simulink model "ControlSystems19"  (R2020b)
settings: Solver=VariableStepAuto  StartTime=0.0  StopTime=100  FixedStep=0.001  MinStep=1e-5
undefined symbols (not defined in the file): DiscIntNeverNeededParam, magnitude
libraries: fl_lib x8, ee_lib x6, nesl_utility x6, pid_lib x5, simulink x3, powerlib x1
(part 1 of 2)
settings Model: Creator=markb  LastModifiedBy=orangejuzi
settings SolverCC: ShapePreserveControl=EnableAll  AlgebraicLoopSolver=LineSearch  MinimalZcImpactIntegration=on
settings DebuggingCC: ReadBeforeWriteMsg=DisableAll  WriteAfterWriteMsg=DisableAll  WriteAfterReadMsg=DisableAll  MaxConsecutiveZCsMsg=warning  MultiTaskDSMMsg=none  ModelReferenceExtraNoncontSigs=warning
settings ModelReferenceCC: UpdateModelReferenceTargets=IfOutOfDate
settings SFSimCC: SFSimEcho=off

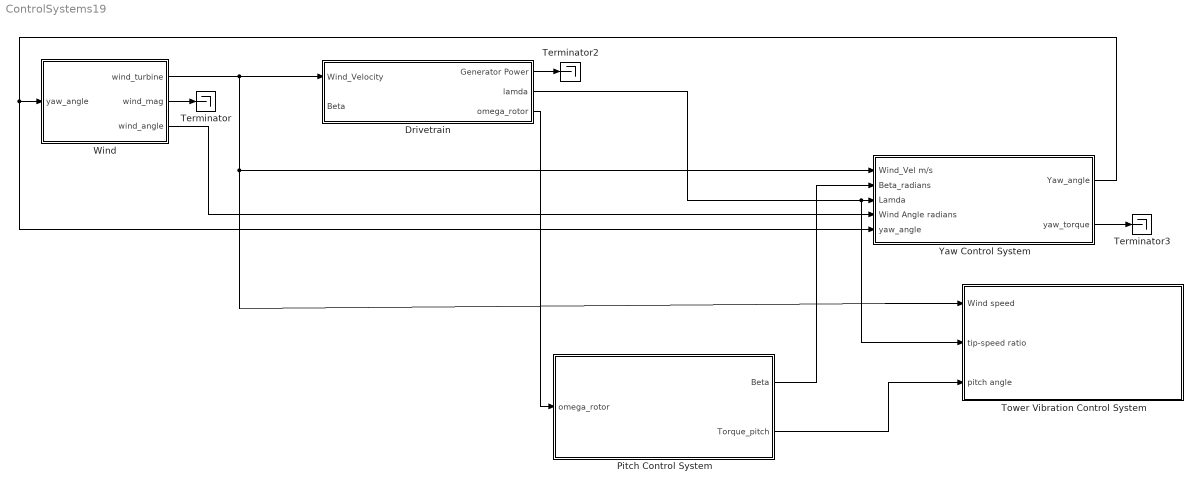
== system ControlSystems19 ==
  Drivetrain : Subsystem
  Pitch Control System : Subsystem
  Terminator : Terminator
  Terminator2 : Terminator
  Terminator3 : Terminator
  Tower Vibration Control System : Subsystem
  Wind : Subsystem
  Yaw Control System : Subsystem
  wires:
  Yaw Control System/1(Yaw_angle) -> Yaw Control System/5(yaw_angle), Wind/1(yaw_angle)
  Wind/2(wind_mag) -> Terminator/1
  Drivetrain/1(Generator Power) -> Terminator2/1
  Wind/3(wind_angle) -> Yaw Control System/4(Wind Angle radians)
  Wind/1(wind_turbine) -> Drivetrain/1(Wind_Velocity), Tower Vibration Control System/1(Wind speed), Yaw Control System/1(Wind_Vel m/s)
  Yaw Control System/2(yaw_torque) -> Terminator3/1
  Drivetrain/2(lamda) -> Tower Vibration Control System/2(tip-speed ratio), Yaw Control System/3(Lamda)
  Drivetrain/3(omega_rotor) -> Pitch Control System/1(omega_rotor)
  Pitch Control System/1(Beta) -> Yaw Control System/2(Beta_radians)
  Pitch Control System/2(Torque_pitch) -> Tower Vibration Control System/3("pitch angle ")

== system ControlSystems19/Drivetrain ==
  Wind_Velocity : Inport
  Beta : Inport  Port=2
  Aerodynamic Block : Subsystem
  Electricl Block : Subsystem
  Mechanical Bock : Subsystem
  Generator Power : Outport
  lamda : Outport  Port=2
  omega_rotor : Outport  Port=3
  wires:
  Mechanical Bock/2(omega_Gen) -> Electricl Block/1(HSS_Speed)
  Electricl Block/2(Generator Torque) -> Mechanical Bock/2(Gen_Torque)
  Mechanical Bock/1(omega_rotor) -> omega_rotor/1, Aerodynamic Block/1(Rotor_Angular_Velocity)
  Wind_Velocity/1 -> Aerodynamic Block/2(Wind_Velocity)
  Beta/1 -> Aerodynamic Block/3(Beta)
  Aerodynamic Block/2(lamda) -> lamda/1
  Aerodynamic Block/1(Rotor_Torque) -> Mechanical Bock/1(Rotor_Torque)
  Electricl Block/1(Generator Power) -> Generator Power/1

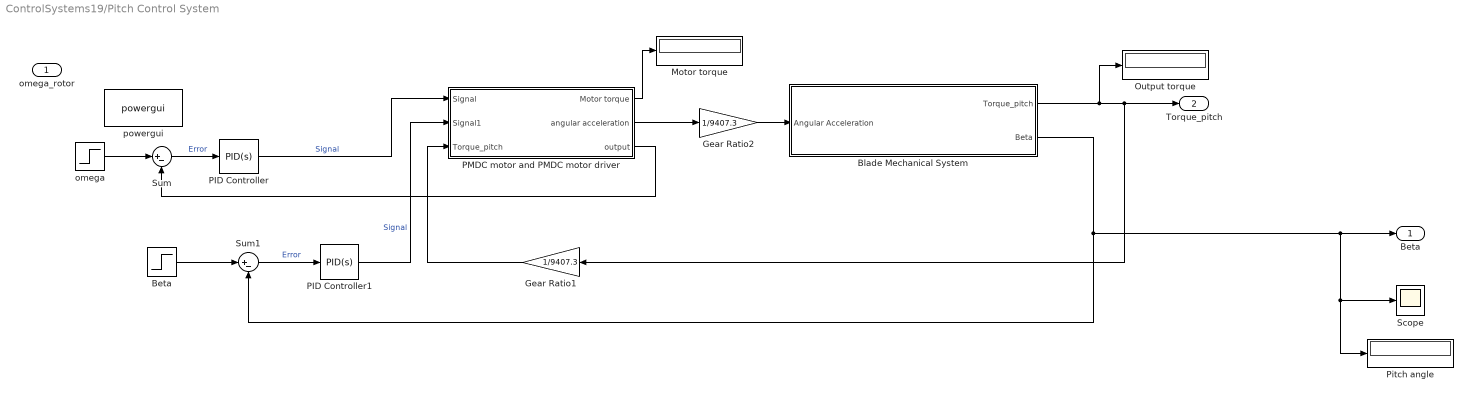
== system ControlSystems19/Pitch Control System ==
  omega_rotor : Inport
  " Beta " : Step  After=0.2976  SampleTime=0
  " omega" : Step  After=2.017  SampleTime=0
  Blade Mechanical System : Subsystem
  Gear Ratio1 : Gain  Gain=1/9407.3
  Gear Ratio2 : Gain  Gain=1/9407.3
  Motor torque : Display
  Output torque : Display
  PID Controller : pid_lib/PID Controller  Controller=PID  Form=Parallel  TimeDomain=Continuous-time  UseExternalTs=off  SampleTime=-1  IntegratorMethod=Forward Euler  FilterMethod=Forward Euler  ControllerParametersSource=internal  P=1  I=1  D=0  UseFilter=on  N=100  TunerSelectOption=Transfer Function Based (PID Tuner App)  InitialConditionSource=internal  InitialConditionForIntegrator=0  InitialConditionForFilter=0  DifferentiatorICPrevScaledInput=0  ExternalReset=none  TrackingMode=off  Kt=1  LimitOutput=off  SatLimitsSource=internal  UpperSaturationLimit=inf  LowerSaturationLimit=-inf  LinearizeAsGain=on  AntiWindupMode=none  Kb=1  POutMin=[]  POutMax=[]  IOutMin=[]  IOutMax=[]  DOutMin=[]  DOutMax=[]  NOutMin=[]  NOutMax=[]  SumOutMin=[]  SumOutMax=[]  SaturationOutMin=[]  SaturationOutMax=[]  PParamMin=[]  PParamMax=[]  IParamMin=[]  IParamMax=[]  DParamMin=[]  DParamMax=[]  NParamMin=[]  NParamMax=[]  KbParamMin=[]  KbParamMax=[]  KtParamMin=[]  KtParamMax=[]  KbOutMin=[]  KbOutMax=[]  KtOutMin=[]  KtOutMax=[]  IntegratorOutMin=[]  IntegratorOutMax=[]  FilterOutMin=[]  FilterOutMax=[]  SumI1OutMin=[]  SumI1OutMax=[]  SumI2OutMin=[]  SumI2OutMax=[]  SumI3OutMin=[]  SumI3OutMax=[]  SumI4OutMin=[]  SumI4OutMax=[]  SumDOutMin=[]  SumDOutMax=[]  DifferentiatorOutMin=[]  DifferentiatorOutMax=[]  FilterDiffOutCoefMin=[]  FilterDiffOutCoefMax=[]  ReciprocalOutMin=[]  ReciprocalOutMax=[]  SumDenOutMin=[]  SumDenOutMax=[]  SumNumOutMin=[]  SumNumOutMax=[]  DivideOutMin=[]  DivideOutMax=[]  UdiffTsProdOutMin=[]  UdiffTsProdOutMax=[]  NTsProdOutMin=[]  NTsProdOutMax=[]  UintegralTsProdOutMin=[]  UintegralTsProdOutMax=[]  UngainTsProdOutMin=[]  UngainTsProdOutMax=[]  IntegratorContinuousStateAttributes=''  IntegratorStateMustResolveToSignalObject=off  IntegratorRTWStateStorageClass=Auto  FilterContinuousStateAttributes=''  FilterStateMustResolveToSignalObject=off  FilterRTWStateStorageClass=Auto  ParallelPVariant=InternalParameters  IdealPVariant=Disabled  IVariant=InternalParameters  DVariant=InternalParameters  IntegratorVariant=Continuous  SatVariant=Disabled  AWVariant=Passthrough  PCopyVariant=Disabled  TRVariant=Disabled  FdbkBlocksVariant=Forward  IdealPFdbkVariant=Disabled  SatFdbkVariant=Disabled  DerivativeFilterVariant=ContFilter  NVariant=InternalParameters  NCopyVariant=Disabled  FilterICVariant=InternalICsFilter  IntegratorICVariant=InternalICs  ExternalResetVariant=Disabled  TRSumVariant=Passthrough  SumFdbkVariant=Disabled  SumVariant=Sum_PID  TsampFilterVariant=InternalTs  TsampNgainVariant=Passthrough  TsampIntegralVariant=Passthrough  ExternalSaturationOutDataTypeStr=Inherit: Same as second input
  PID Controller1 : pid_lib/PID Controller  Controller=PID  Form=Parallel  TimeDomain=Continuous-time  UseExternalTs=off  SampleTime=-1  IntegratorMethod=Forward Euler  FilterMethod=Forward Euler  ControllerParametersSource=internal  P=1  I=1  D=0  UseFilter=on  N=100  TunerSelectOption=Transfer Function Based (PID Tuner App)  InitialConditionSource=internal  InitialConditionForIntegrator=0  InitialConditionForFilter=0  DifferentiatorICPrevScaledInput=0  ExternalReset=none  TrackingMode=off  Kt=1  LimitOutput=off  SatLimitsSource=internal  UpperSaturationLimit=inf  LowerSaturationLimit=-inf  LinearizeAsGain=on  AntiWindupMode=none  Kb=1  POutMin=[]  POutMax=[]  IOutMin=[]  IOutMax=[]  DOutMin=[]  DOutMax=[]  NOutMin=[]  NOutMax=[]  SumOutMin=[]  SumOutMax=[]  SaturationOutMin=[]  SaturationOutMax=[]  PParamMin=[]  PParamMax=[]  IParamMin=[]  IParamMax=[]  DParamMin=[]  DParamMax=[]  NParamMin=[]  NParamMax=[]  KbParamMin=[]  KbParamMax=[]  KtParamMin=[]  KtParamMax=[]  KbOutMin=[]  KbOutMax=[]  KtOutMin=[]  KtOutMax=[]  IntegratorOutMin=[]  IntegratorOutMax=[]  FilterOutMin=[]  FilterOutMax=[]  SumI1OutMin=[]  SumI1OutMax=[]  SumI2OutMin=[]  SumI2OutMax=[]  SumI3OutMin=[]  SumI3OutMax=[]  SumI4OutMin=[]  SumI4OutMax=[]  SumDOutMin=[]  SumDOutMax=[]  DifferentiatorOutMin=[]  DifferentiatorOutMax=[]  FilterDiffOutCoefMin=[]  FilterDiffOutCoefMax=[]  ReciprocalOutMin=[]  ReciprocalOutMax=[]  SumDenOutMin=[]  SumDenOutMax=[]  SumNumOutMin=[]  SumNumOutMax=[]  DivideOutMin=[]  DivideOutMax=[]  UdiffTsProdOutMin=[]  UdiffTsProdOutMax=[]  NTsProdOutMin=[]  NTsProdOutMax=[]  UintegralTsProdOutMin=[]  UintegralTsProdOutMax=[]  UngainTsProdOutMin=[]  UngainTsProdOutMax=[]  IntegratorContinuousStateAttributes=''  IntegratorStateMustResolveToSignalObject=off  IntegratorRTWStateStorageClass=Auto  FilterContinuousStateAttributes=''  FilterStateMustResolveToSignalObject=off  FilterRTWStateStorageClass=Auto  ParallelPVariant=InternalParameters  IdealPVariant=Disabled  IVariant=InternalParameters  DVariant=InternalParameters  IntegratorVariant=Continuous  SatVariant=Disabled  AWVariant=Passthrough  PCopyVariant=Disabled  TRVariant=Disabled  FdbkBlocksVariant=Forward  IdealPFdbkVariant=Disabled  SatFdbkVariant=Disabled  DerivativeFilterVariant=ContFilter  NVariant=InternalParameters  NCopyVariant=Disabled  FilterICVariant=InternalICsFilter  IntegratorICVariant=InternalICs  ExternalResetVariant=Disabled  TRSumVariant=Passthrough  SumFdbkVariant=Disabled  SumVariant=Sum_PID  TsampFilterVariant=InternalTs  TsampNgainVariant=Passthrough  TsampIntegralVariant=Passthrough  ExternalSaturationOutDataTypeStr=Inherit: Same as second input
  PMDC motor and PMDC motor driver : Subsystem
  Pitch angle : Display
  Scope : Scope
  Sum : Sum  Inputs=|+-
  Sum1 : Sum  Inputs=|+-
  powergui : powerlib/powergui  Priority=1  SimulationMode=Continuous  SampleTime=50e-6  frequency=60  Iterations=50  frequencyindice=0  Pbase=100e6  ErrMax=1e-4  UnitsV=kV  UnitsW=MW  buscounter=0  FunctionMessages=off  echomessages=off  EnableUseOfTLC=off  CurrentSourceSwitches=off  DisableSnubberDevices=off  DisableRonSwitches=off  DisableVfSwitches=off  DisplayEquations=off  AutomaticDiscreteSolvers=off  SolverType=Tustin/Backward Euler (TBE)  Interpol=off  ExternalGateDelay=off  methode=off  Ts=100  x0status=blocks  SPID=on  SwTol=0  HookPort=off  NonlinearTolerance=1e-4  nMaxIteration=100  ContinueOnMaxIteration=off  RestoreLinks=warning  ResistiveCurrentMeasurement=off  Frange=[0:2:500]  Ylog=off  Xlog=on  ShowGrid=off  save=off  variable=ZData  structure=0  ZoomFFT=off  StartTime=0.0  cycles=1  DisplayStyle=1  fundamental=60  FreqAxis=off  MaxFrequency=1000  frequencyindicesteady=1  RmsSteady=1  display=off
  Beta : Outport
  Torque_pitch : Outport  Port=2
  wires:
  Sum1/1 -> PID Controller1/1  "Error"
  Blade Mechanical System/2(Beta) -> Beta/1, Scope/1, Pitch angle/1, Sum1/2
  " omega"/1 -> Sum/1
  " Beta "/1 -> Sum1/1
  Sum/1 -> PID Controller/1  "Error"
  PMDC motor and PMDC motor driver/3(output) -> Sum/2
  PMDC motor and PMDC motor driver/2(angular acceleration) -> Gear Ratio2/1
  PMDC motor and PMDC motor driver/1(Motor torque) -> Motor torque/1
  Gear Ratio1/1 -> PMDC motor and PMDC motor driver/3(Torque_pitch)
  Blade Mechanical System/1(Torque_pitch) -> Gear Ratio1/1, Torque_pitch/1, Output torque/1
  PID Controller/1 -> PMDC motor and PMDC motor driver/1(Signal)  "Signal"
  PID Controller1/1 -> PMDC motor and PMDC motor driver/2(Signal1)  "Signal"
  Gear Ratio2/1 -> Blade Mechanical System/1(Angular Acceleration)

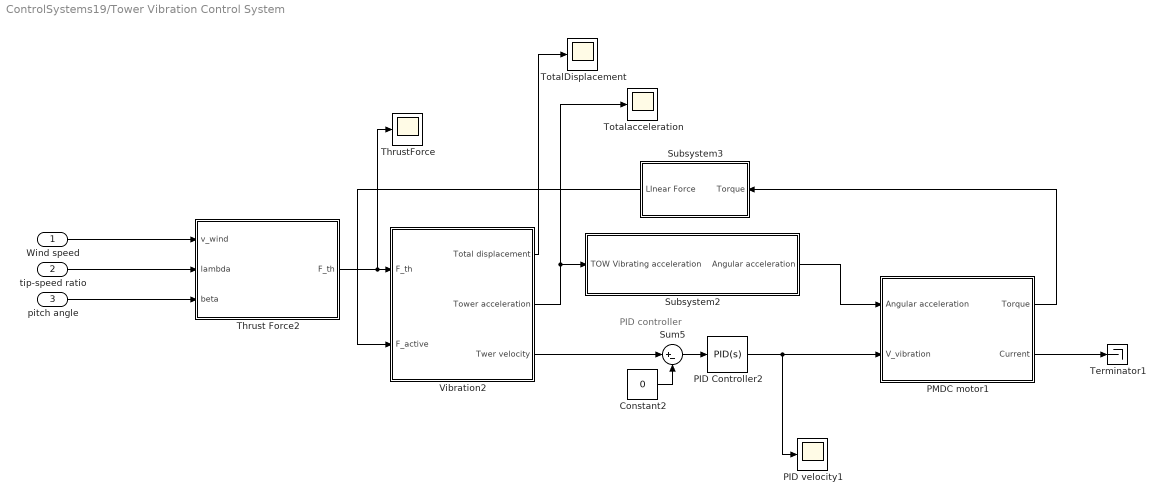
== system ControlSystems19/Tower Vibration Control System ==
  note: PID controller
  Wind speed : Inport
  tip-speed ratio : Inport  Port=2
  "pitch angle " : Inport  Port=3
  Constant2 : Constant  Value=0
  PID Controller2 : pid_lib/PID Controller  Controller=PID  Form=Parallel  TimeDomain=Continuous-time  UseExternalTs=off  SampleTime=-1  IntegratorMethod=Forward Euler  FilterMethod=Forward Euler  ControllerParametersSource=internal  P=-253332.952785958  I=-6447426.88773076  D=723.347381885761  UseFilter=on  N=350.223086624743  TunerSelectOption=Transfer Function Based (PID Tuner App)  InitialConditionSource=internal  InitialConditionForIntegrator=0  InitialConditionForFilter=0  DifferentiatorICPrevScaledInput=0  ExternalReset=none  TrackingMode=off  Kt=1  LimitOutput=off  SatLimitsSource=internal  UpperSaturationLimit=inf  LowerSaturationLimit=-inf  LinearizeAsGain=on  AntiWindupMode=none  Kb=1  POutMin=[]  POutMax=[]  IOutMin=[]  IOutMax=[]  DOutMin=[]  DOutMax=[]  NOutMin=[]  NOutMax=[]  SumOutMin=[]  SumOutMax=[]  SaturationOutMin=[]  SaturationOutMax=[]  PParamMin=[]  PParamMax=[]  IParamMin=[]  IParamMax=[]  DParamMin=[]  DParamMax=[]  NParamMin=[]  NParamMax=[]  KbParamMin=[]  KbParamMax=[]  KtParamMin=[]  KtParamMax=[]  KbOutMin=[]  KbOutMax=[]  KtOutMin=[]  KtOutMax=[]  IntegratorOutMin=[]  IntegratorOutMax=[]  FilterOutMin=[]  FilterOutMax=[]  SumI1OutMin=[]  SumI1OutMax=[]  SumI2OutMin=[]  SumI2OutMax=[]  SumI3OutMin=[]  SumI3OutMax=[]  SumI4OutMin=[]  SumI4OutMax=[]  SumDOutMin=[]  SumDOutMax=[]  DifferentiatorOutMin=[]  DifferentiatorOutMax=[]  FilterDiffOutCoefMin=[]  FilterDiffOutCoefMax=[]  ReciprocalOutMin=[]  ReciprocalOutMax=[]  SumDenOutMin=[]  SumDenOutMax=[]  SumNumOutMin=[]  SumNumOutMax=[]  DivideOutMin=[]  DivideOutMax=[]  UdiffTsProdOutMin=[]  UdiffTsProdOutMax=[]  NTsProdOutMin=[]  NTsProdOutMax=[]  UintegralTsProdOutMin=[]  UintegralTsProdOutMax=[]  UngainTsProdOutMin=[]  UngainTsProdOutMax=[]  IntegratorContinuousStateAttributes=''  IntegratorStateMustResolveToSignalObject=off  IntegratorRTWStateStorageClass=Auto  FilterContinuousStateAttributes=''  FilterStateMustResolveToSignalObject=off  FilterRTWStateStorageClass=Auto  ParallelPVariant=InternalParameters  IdealPVariant=Disabled  IVariant=InternalParameters  DVariant=InternalParameters  IntegratorVariant=Continuous  SatVariant=Disabled  AWVariant=Passthrough  PCopyVariant=Disabled  TRVariant=Disabled  FdbkBlocksVariant=Forward  IdealPFdbkVariant=Disabled  SatFdbkVariant=Disabled  DerivativeFilterVariant=ContFilter  NVariant=InternalParameters  NCopyVariant=Disabled  FilterICVariant=InternalICsFilter  IntegratorICVariant=InternalICs  ExternalResetVariant=Disabled  TRSumVariant=Passthrough  SumFdbkVariant=Disabled  SumVariant=Sum_PID  TsampFilterVariant=InternalTs  TsampNgainVariant=Passthrough  TsampIntegralVariant=Passthrough  ExternalSaturationOutDataTypeStr=Inherit: Same as second input
  PID velocity1 : Scope
  PMDC motor1 : Subsystem
  Subsystem2 : Subsystem
  Subsystem3 : Subsystem
  Sum5 : Sum  Inputs=|+-
  Terminator1 : Terminator
  Thrust Force2 : Subsystem
  ThrustForce : Scope
  TotalDisplacement : Scope
  Totalacceleration : Scope
  Vibration2 : Subsystem
  wires:
  Wind speed/1 -> Thrust Force2/1(v_wind)
  "pitch angle "/1 -> Thrust Force2/3(beta)
  tip-speed ratio/1 -> Thrust Force2/2(lambda)
  PMDC motor1/2(Current) -> Terminator1/1
  Subsystem2/1(Angular acceleration) -> PMDC motor1/1(Angular acceleration)
  Sum5/1 -> PID Controller2/1
  Constant2/1 -> Sum5/2
  PID Controller2/1 -> PID velocity1/1, PMDC motor1/2(V_vibration)
  PMDC motor1/1(Torque) -> Subsystem3/1(Torque)
  Vibration2/2(Tower acceleration) -> Totalacceleration/1, Subsystem2/1(TOW Vibrating acceleration)
  Thrust Force2/1(F_th) -> ThrustForce/1, Vibration2/1(F_th)
  Vibration2/1(Total displacement) -> TotalDisplacement/1
  Subsystem3/1(LInear Force) -> Vibration2/2(F_active)
  Vibration2/3(Twer velocity) -> Sum5/1

== system ControlSystems19/Wind ==
  yaw_angle : Inport
  Add : Sum  Inputs=-+
  Product : Product
  Ramp_for_wind_test : simulink/Sources/Ramp  slope=0.1  start=0  InitialOutput=10
  Terminator : Terminator
  Trigonometric Function : Trigonometry  Operator=cos
  Wind_mag : simulink/Sources/Repeating Sequence Interpolated  OutValues=[6 10 15 10 10 15 18 20 22 26 20 22 18 15 13 13 12 10 9 11 17 17 19 19 25 25 26 19 13 10 7 ].'  TimeValues=[0 5 15 20 25 30 35 40 45 50 55 60 65 70 75 80 85 90 95 100 105 110 115 120 125 130 135 140 145 150 155 ].'  LookUpMeth=Interpolation-Use End Values  tsamp=0.01  OutMin=[]  OutMax=[]  OutDataTypeStr=double  OutputDataTypeScalingMode=double  OutDataType=fixdt(0,8)  OutScaling=2^-10
  deg_to_rad : Gain  Gain=pi/180
  omega_w_deg : simulink/Sources/Repeating Sequence Interpolated  OutValues=[ 0 0 0 6 10 12 12 4 8 12 16 16 24 28 24 16 12 4 2 0 0 -2 -4 -4 -10 -14 -18 -20 -12 -8 -4 ].'  TimeValues=[0 5 15 20 25 30 35 40 45 50 55 60 65 70 75 80 85 90 95 100 105 110 115 120 125 130 135 140 145 150 155 ].'  LookUpMeth=Interpolation-Use End Values  tsamp=0.01  OutMin=[]  OutMax=[]  OutDataTypeStr=double  OutputDataTypeScalingMode=double  OutDataType=fixdt(0,8)  OutScaling=2^-10
  wind_turbine : Outport
  wind_mag : Outport  Port=2
  wind_angle : Outport  Port=3
  wires:
  Add/1 -> Trigonometric Function/1
  Trigonometric Function/1 -> Product/1
  deg_to_rad/1 -> wind_angle/1, Add/2
  yaw_angle/1 -> Add/1
  omega_w_deg/1 -> deg_to_rad/1
  Wind_mag/1 -> wind_mag/1, Product/2
  Product/1 -> wind_turbine/1
  Ramp_for_wind_test/1 -> Terminator/1

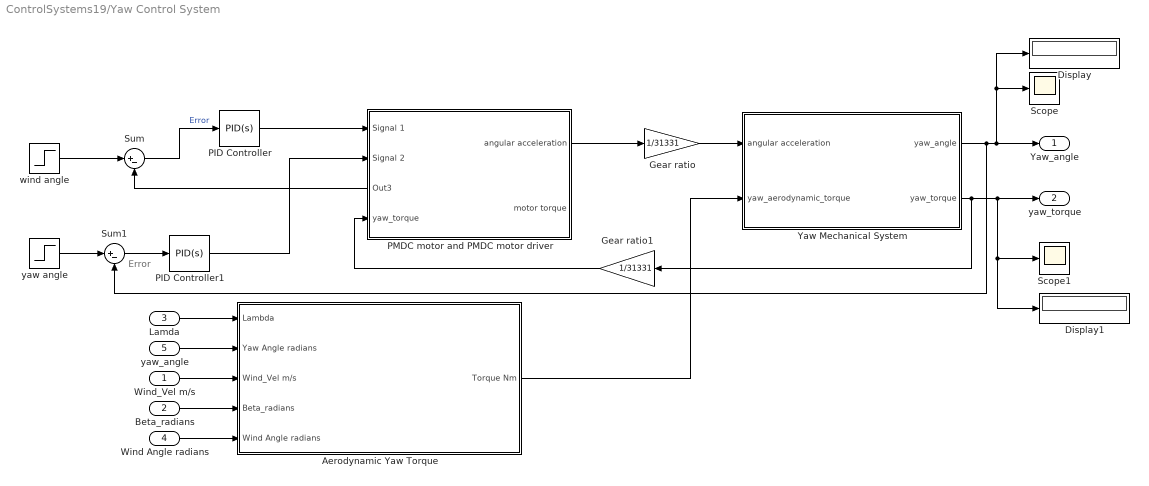
== system ControlSystems19/Yaw Control System ==
  note: Error
  Wind_Vel m/s : Inport
  Beta_radians : Inport  Port=2
  Lamda : Inport  Port=3
  Wind Angle radians : Inport  Port=4
  yaw_angle : Inport  Port=5
  Aerodynamic Yaw Torque : Subsystem
  Display : Display
  Display1 : Display
  Gear ratio : Gain  Gain=1/31331
  Gear ratio1 : Gain  Gain=1/31331
  PID Controller : pid_lib/PID Controller  Controller=PID  Form=Parallel  TimeDomain=Continuous-time  UseExternalTs=off  SampleTime=-1  IntegratorMethod=Forward Euler  FilterMethod=Forward Euler  ControllerParametersSource=internal  P=1  I=1  D=1  UseFilter=on  N=100  TunerSelectOption=Transfer Function Based (PID Tuner App)  InitialConditionSource=internal  InitialConditionForIntegrator=0  InitialConditionForFilter=0  DifferentiatorICPrevScaledInput=0  ExternalReset=none  TrackingMode=off  Kt=1  LimitOutput=off  SatLimitsSource=internal  UpperSaturationLimit=inf  LowerSaturationLimit=-inf  LinearizeAsGain=on  AntiWindupMode=none  Kb=1  POutMin=[]  POutMax=[]  IOutMin=[]  IOutMax=[]  DOutMin=[]  DOutMax=[]  NOutMin=[]  NOutMax=[]  SumOutMin=[]  SumOutMax=[]  SaturationOutMin=[]  SaturationOutMax=[]  PParamMin=[]  PParamMax=[]  IParamMin=[]  IParamMax=[]  DParamMin=[]  DParamMax=[]  NParamMin=[]  NParamMax=[]  KbParamMin=[]  KbParamMax=[]  KtParamMin=[]  KtParamMax=[]  KbOutMin=[]  KbOutMax=[]  KtOutMin=[]  KtOutMax=[]  IntegratorOutMin=[]  IntegratorOutMax=[]  FilterOutMin=[]  FilterOutMax=[]  SumI1OutMin=[]  SumI1OutMax=[]  SumI2OutMin=[]  SumI2OutMax=[]  SumI3OutMin=[]  SumI3OutMax=[]  SumI4OutMin=[]  SumI4OutMax=[]  SumDOutMin=[]  SumDOutMax=[]  DifferentiatorOutMin=[]  DifferentiatorOutMax=[]  FilterDiffOutCoefMin=[]  FilterDiffOutCoefMax=[]  ReciprocalOutMin=[]  ReciprocalOutMax=[]  SumDenOutMin=[]  SumDenOutMax=[]  SumNumOutMin=[]  SumNumOutMax=[]  DivideOutMin=[]  DivideOutMax=[]  UdiffTsProdOutMin=[]  UdiffTsProdOutMax=[]  NTsProdOutMin=[]  NTsProdOutMax=[]  UintegralTsProdOutMin=[]  UintegralTsProdOutMax=[]  UngainTsProdOutMin=[]  UngainTsProdOutMax=[]  IntegratorContinuousStateAttributes=''  IntegratorStateMustResolveToSignalObject=off  IntegratorRTWStateStorageClass=Auto  FilterContinuousStateAttributes=''  FilterStateMustResolveToSignalObject=off  FilterRTWStateStorageClass=Auto  ParallelPVariant=InternalParameters  IdealPVariant=Disabled  IVariant=InternalParameters  DVariant=InternalParameters  IntegratorVariant=Continuous  SatVariant=Disabled  AWVariant=Passthrough  PCopyVariant=Disabled  TRVariant=Disabled  FdbkBlocksVariant=Forward  IdealPFdbkVariant=Disabled  SatFdbkVariant=Disabled  DerivativeFilterVariant=ContFilter  NVariant=InternalParameters  NCopyVariant=Disabled  FilterICVariant=InternalICsFilter  IntegratorICVariant=InternalICs  ExternalResetVariant=Disabled  TRSumVariant=Passthrough  SumFdbkVariant=Disabled  SumVariant=Sum_PID  TsampFilterVariant=InternalTs  TsampNgainVariant=Passthrough  TsampIntegralVariant=Passthrough  ExternalSaturationOutDataTypeStr=Inherit: Same as second input
  PID Controller1 : pid_lib/PID Controller  Controller=PID  Form=Parallel  TimeDomain=Continuous-time  UseExternalTs=off  SampleTime=-1  IntegratorMethod=Forward Euler  FilterMethod=Forward Euler  ControllerParametersSource=internal  P=1  I=1  D=0  UseFilter=on  N=100  TunerSelectOption=Transfer Function Based (PID Tuner App)  InitialConditionSource=internal  InitialConditionForIntegrator=0  InitialConditionForFilter=0  DifferentiatorICPrevScaledInput=0  ExternalReset=none  TrackingMode=off  Kt=1  LimitOutput=off  SatLimitsSource=internal  UpperSaturationLimit=inf  LowerSaturationLimit=-inf  LinearizeAsGain=on  AntiWindupMode=none  Kb=1  POutMin=[]  POutMax=[]  IOutMin=[]  IOutMax=[]  DOutMin=[]  DOutMax=[]  NOutMin=[]  NOutMax=[]  SumOutMin=[]  SumOutMax=[]  SaturationOutMin=[]  SaturationOutMax=[]  PParamMin=[]  PParamMax=[]  IParamMin=[]  IParamMax=[]  DParamMin=[]  DParamMax=[]  NParamMin=[]  NParamMax=[]  KbParamMin=[]  KbParamMax=[]  KtParamMin=[]  KtParamMax=[]  KbOutMin=[]  KbOutMax=[]  KtOutMin=[]  KtOutMax=[]  IntegratorOutMin=[]  IntegratorOutMax=[]  FilterOutMin=[]  FilterOutMax=[]  SumI1OutMin=[]  SumI1OutMax=[]  SumI2OutMin=[]  SumI2OutMax=[]  SumI3OutMin=[]  SumI3OutMax=[]  SumI4OutMin=[]  SumI4OutMax=[]  SumDOutMin=[]  SumDOutMax=[]  DifferentiatorOutMin=[]  DifferentiatorOutMax=[]  FilterDiffOutCoefMin=[]  FilterDiffOutCoefMax=[]  ReciprocalOutMin=[]  ReciprocalOutMax=[]  SumDenOutMin=[]  SumDenOutMax=[]  SumNumOutMin=[]  SumNumOutMax=[]  DivideOutMin=[]  DivideOutMax=[]  UdiffTsProdOutMin=[]  UdiffTsProdOutMax=[]  NTsProdOutMin=[]  NTsProdOutMax=[]  UintegralTsProdOutMin=[]  UintegralTsProdOutMax=[]  UngainTsProdOutMin=[]  UngainTsProdOutMax=[]  IntegratorContinuousStateAttributes=''  IntegratorStateMustResolveToSignalObject=off  IntegratorRTWStateStorageClass=Auto  FilterContinuousStateAttributes=''  FilterStateMustResolveToSignalObject=off  FilterRTWStateStorageClass=Auto  ParallelPVariant=InternalParameters  IdealPVariant=Disabled  IVariant=InternalParameters  DVariant=InternalParameters  IntegratorVariant=Continuous  SatVariant=Disabled  AWVariant=Passthrough  PCopyVariant=Disabled  TRVariant=Disabled  FdbkBlocksVariant=Forward  IdealPFdbkVariant=Disabled  SatFdbkVariant=Disabled  DerivativeFilterVariant=ContFilter  NVariant=InternalParameters  NCopyVariant=Disabled  FilterICVariant=InternalICsFilter  IntegratorICVariant=InternalICs  ExternalResetVariant=Disabled  TRSumVariant=Passthrough  SumFdbkVariant=Disabled  SumVariant=Sum_PID  TsampFilterVariant=InternalTs  TsampNgainVariant=Passthrough  TsampIntegralVariant=Passthrough  ExternalSaturationOutDataTypeStr=Inherit: Same as second input
  PMDC motor and PMDC motor driver : Subsystem
      settings: PortSchema="{\"entries\":[{\"content\":{\"sides\":[{\"content\":{\"connectorIds\":[\"In1\",\"In2\",\"Out3\",\"In3\"]},\"type\":\"ConnectorPlacement.EquallySpacedRectSide\",\"uuid\":\"28067f50-3c14-4cc3-b57d-002bf70ae05c\"},{\"content\":{\"connectorIds\":[\"Out1\",\"Out2\"],\"side\":\"RIGHT\"},\"type\":\"ConnectorPlacement.EquallySpacedRectSide\",\"uuid\":\"1f2ec377-fb05-461e-9b84-5db73f33a164\"},{\"content\":{\"connectorIds\":[],\"side\":\"TOP\"},\"type\":\"ConnectorPlacement.EquallySpacedRectSide\",\"uuid\":\"ac3ec224-c2fb-4581-a86f-0922aa74f226\"},{\"content\":{\"connectorIds\":[],\"side\":\"HIDDEN\"},\"type\":\"ConnectorPlacement.EquallySpacedRectSide\",\"uuid\":\"3e076245-2eb8-43f8-b3f5-02876c6856f1\"}]},\"type\":\"ConnectorPlacement.EquallySpacedConnector\",\"uuid\":\"3cc3f2e2-a5c0-4020-b3af-0be15bb2ba6f\"}],\"packageUris\":[\"http://schema.mathworks.com/mf0/Connector/R2020b\"],\"version\":\"1.0\"}"
  Scope : Scope
  Scope1 : Scope
  Sum : Sum  Inputs=|+-
  Sum1 : Sum  Inputs=|+-
  Yaw Mechanical System : Subsystem
  wind angle : Step  SampleTime=0
  yaw angle : Step  SampleTime=0
  Yaw_angle : Outport
  yaw_torque : Outport  Port=2
  wires:
  Wind_Vel m/s/1 -> Aerodynamic Yaw Torque/3(Wind_Vel m/s)
  Wind Angle radians/1 -> Aerodynamic Yaw Torque/5(Wind Angle radians)
  Beta_radians/1 -> Aerodynamic Yaw Torque/4(Beta_radians)
  Lamda/1 -> Aerodynamic Yaw Torque/1(Lambda)
  Aerodynamic Yaw Torque/1(Torque Nm) -> Yaw Mechanical System/2(yaw_aerodynamic_torque)
  yaw_angle/1 -> Aerodynamic Yaw Torque/2(Yaw Angle radians)
  Yaw Mechanical System/2(yaw_torque) -> Scope1/1, Display1/1, yaw_torque/1, Gear ratio1/1
  Yaw Mechanical System/1(yaw_angle) -> Sum1/2, Yaw_angle/1, Display/1, Scope/1
  Gear ratio/1 -> Yaw Mechanical System/1(angular acceleration)
  PID Controller1/1 -> PMDC motor and PMDC motor driver/2(Signal 2)
  PID Controller/1 -> PMDC motor and PMDC motor driver/1(Signal 1)
  Sum1/1 -> PID Controller1/1
  wind angle/1 -> Sum/1
  PMDC motor and PMDC motor driver/3(Out3) -> Sum/2
  Sum/1 -> PID Controller/1  "Error"
  yaw angle/1 -> Sum1/1
  PMDC motor and PMDC motor driver/1(angular acceleration) -> Gear ratio/1
  Gear ratio1/1 -> PMDC motor and PMDC motor driver/3(yaw_torque)

== system ControlSystems19/Drivetrain/Aerodynamic Block ==
  Rotor_Angular_Velocity : Inport
  Wind_Velocity : Inport  Port=2
  Beta : Inport  Port=3
  Power Coefficient : Subsystem
  Rotor Torque : Subsystem
  Tip speed Ratio : Subsystem
  Rotor_Torque : Outport
  lamda : Outport  Port=2
  wires:
  Beta/1 -> Power Coefficient/2(Beta)
  Tip speed Ratio/1(Tip_Speed_Ratio) -> lamda/1, Power Coefficient/1(Lamda)
  Power Coefficient/1(C_p) -> Rotor Torque/1(Power_Coefficient)
  Rotor_Angular_Velocity/1 -> Rotor Torque/3(Rotor_Angular_Velocity), Tip speed Ratio/1(Rotor_Angular_Velocity)
  Rotor Torque/1(Rotor_Torque) -> Rotor_Torque/1
  Wind_Velocity/1 -> Rotor Torque/2(Wind_Speed), Tip speed Ratio/2(Wind_Velocity)

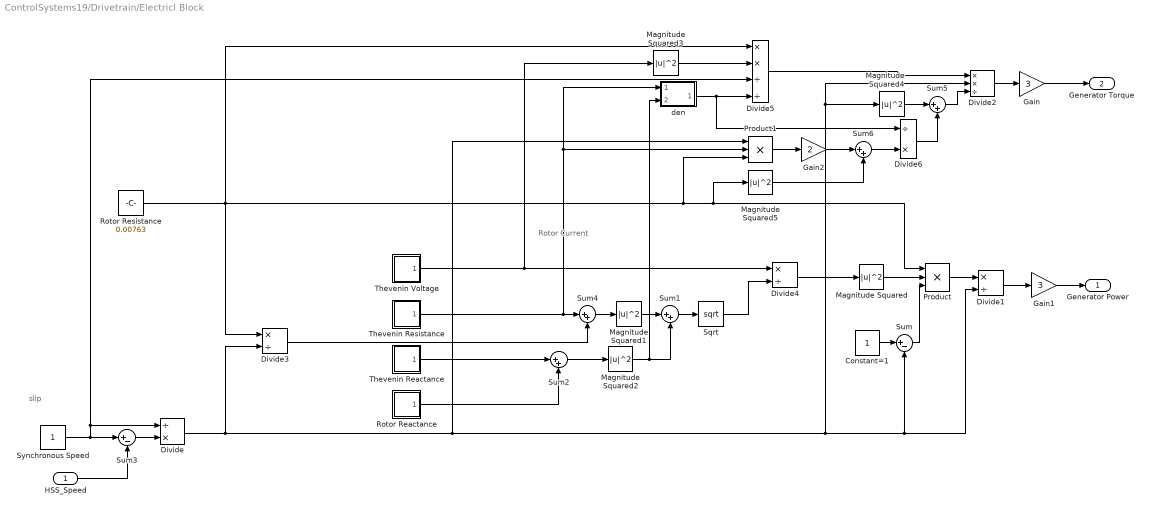
== system ControlSystems19/Drivetrain/Electricl Block ==
  note: slip
  note: Rotor Current
  HSS_Speed : Inport
  Constant=1 : Constant
  Divide : Product  Inputs=/*
  Divide1 : Product  Inputs=*/
  Divide2 : Product  Inputs=**/
  Divide3 : Product  Inputs=*/
  Divide4 : Product  Inputs=*/
  Divide5 : Product  Inputs=**//
  Divide6 : Product  Inputs=/*
  Gain : Gain  Gain=3
  Gain1 : Gain  Gain=3
  Gain2 : Gain  Gain=2
  Magnitude Squared{,1..5} (6 alike) : Math  Operator=magnitude^2  SaturateOnIntegerOverflow=on
  Product : Product  Inputs=3
  Product1 : Product  Inputs=3
  Rotor Reactance : Subsystem
  Rotor Resistance : Constant  Value=0.00763
  Sqrt : Sqrt  SaturateOnIntegerOverflow=on
  Sum : Sum  Inputs=|+-
  Sum{1..2,4..6} (5 alike) : Sum  Inputs=|++
  Sum3 : Sum  Inputs=|+-
  Synchronous Speed : Constant
  Thevenin Reactance : Subsystem
  Thevenin Resistance : Subsystem
  Thevenin Voltage : Subsystem
  den : Subsystem
  Generator Power : Outport
  Generator Torque : Outport  Port=2
  wires:
  Product/1 -> Divide1/1
  Divide1/1 -> Gain1/1
  Gain1/1 -> Generator Power/1
  Sum/1 -> Product/3
  Divide/1 -> Product1/1, Divide1/2, Sum/2, Magnitude Squared4/1, Divide2/2, Divide3/2
  Constant=1/1 -> Sum/1
  Rotor Resistance/1 -> Product1/3, Product/1, Magnitude Squared5/1, Divide3/1, Divide5/1
  Divide4/1 -> Magnitude Squared/1
  Magnitude Squared/1 -> Product/2
  Gain/1 -> Generator Torque/1
  Divide2/1 -> Gain/1
  Thevenin Voltage/1(Out1) -> Magnitude Squared3/1, Divide4/1
  Divide3/1 -> Sum4/2
  Magnitude Squared2/1 -> Sum1/2, den/2(In2)
  Magnitude Squared1/1 -> Sum1/1
  Sqrt/1 -> Divide4/2
  Sum2/1 -> Magnitude Squared2/1
  Thevenin Reactance/1(Out1) -> Sum2/1
  Sum1/1 -> Sqrt/1
  Magnitude Squared3/1 -> Divide5/2
  Synchronous Speed/1 -> Divide5/3, Divide/1, Sum3/1
  HSS_Speed/1 -> Sum3/2
  Sum3/1 -> Divide/2
  Divide5/1 -> Divide2/1
  den/1(Out1) -> Divide6/1, Divide5/4
  Sum4/1 -> Magnitude Squared1/1
  Sum5/1 -> Divide2/3
  Magnitude Squared4/1 -> Sum5/1
  Divide6/1 -> Sum5/2
  Sum6/1 -> Divide6/2
  Gain2/1 -> Sum6/1
  Product1/1 -> Gain2/1
  Magnitude Squared5/1 -> Sum6/2
  Rotor Reactance/1(Out1) -> Sum2/2
  Thevenin Resistance/1(Out1) -> Sum4/1, Product1/2, den/1(In1)

== system ControlSystems19/Drivetrain/Mechanical Bock ==
  Rotor_Torque : Inport
  Gen_Torque : Inport  Port=2
  Discrete-Time Integrator : DiscreteIntegrator  InitialCondition=1.9  SampleTime=-1  ICPrevOutput=DiscIntNeverNeededParam  ICPrevScaledInput=DiscIntNeverNeededParam
  Gain1 : Gain  Gain=1/(2953248+56.442/80^2)
  Gain2 : Gain  Gain=(2953248-56.442*80^2)/(10-1.6*80^2)
  Gear ratio1 : Gain  Gain=80
  Scope : Scope
  Sum : Sum  Inputs=|+--
  omega_rotor : Outport
  omega_Gen : Outport  Port=2
  wires:
  Rotor_Torque/1 -> Sum/1
  Gen_Torque/1 -> Sum/2
  Gain2/1 -> Sum/3
  Gear ratio1/1 -> omega_Gen/1
  Discrete-Time Integrator/1 -> omega_rotor/1, Scope/1, Gear ratio1/1, Gain2/1
  Sum/1 -> Gain1/1
  Gain1/1 -> Discrete-Time Integrator/1

== system ControlSystems19/Pitch Control System/Blade Mechanical System ==
  Angular Acceleration : Inport
  Add1 : Sum  Inputs=+--
  D : Gain  Gain=100
  Integrator6 : Integrator
  Integrator7 : Integrator
  J : Gain  Gain=22800
  T_pitchA2 : Constant  Value=15000
  Torque_pitch : Outport
  Beta : Outport  Port=2
  wires:
  J/1 -> Add1/1
  D/1 -> Add1/2
  T_pitchA2/1 -> Add1/3
  Integrator6/1 -> Integrator7/1, D/1
  Add1/1 -> Torque_pitch/1
  Angular Acceleration/1 -> J/1, Integrator6/1
  Integrator7/1 -> Beta/1

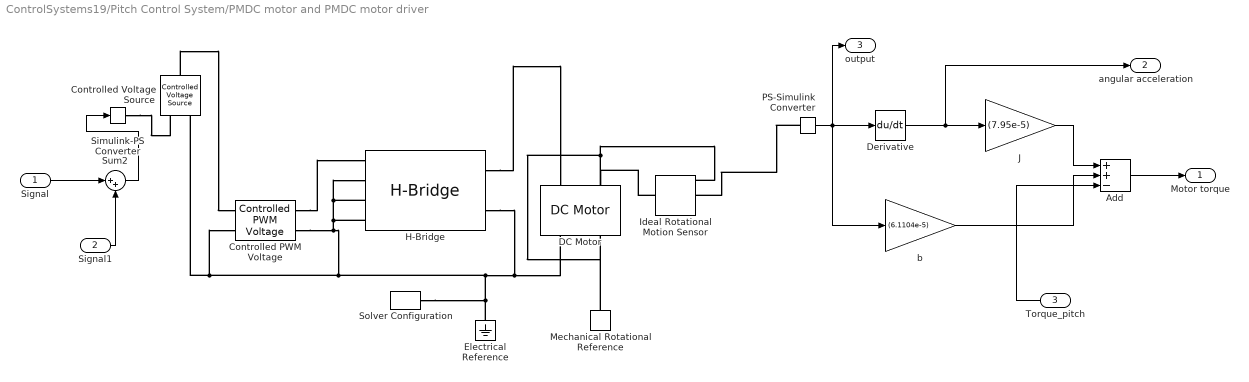
== system ControlSystems19/Pitch Control System/PMDC motor and PMDC motor driver ==
  Signal : Inport
  Signal1 : Inport  Port=2
  Torque_pitch : Inport  Port=3
  Add : Sum  Inputs=++-
  Controlled PWM Voltage : ee_lib/Integrated Circuits/Controlled PWM Voltage  F=1000 Hz  TD=0 s  pulse_width_offset=0 s  pulse_min=0 s  Vmin=0 V  Vmax=5 V  Vm=48 V  pwm_or_av=1  event_type=1  sample_time=1e-6 s  u_min=0  u_max=1
  Controlled Voltage Source : fl_lib/Electrical/Electrical Sources/Controlled Voltage Source
  DC Motor : ee_lib/Electromechanical/Brushed Motors/DC Motor  field_option=ee.enum.field_option.pm  Rf=100 Ohm  Lf=1 H  Laf=0.15 H  If0=0 A  parameterization=ee.enum.dcparam_option.circuit_param  Ra=2.2 Ohm  La=4.681e-3 H  emf_or_torque=ee.enum.emf_or_torque.kv  Kv=0.12 V/(rad/s)  Ki=6.876e-4 N*m/A  T_stall=0.24e-3 N*m  w_max=19100 rpm  w_rated=15000 rpm  P_rated=0.08 W  V_rated=1.5 V  J=7.95e-5 kg*m^2  lam_param=ee.enum.lam_param.damping  lam=6.1104e-5 N*m/(rad/s)  i_noload=0 A  V_i_noload=1.5 V  speed0=0 rad/s  enable_fault_armature=ee.enum.faults.faultEnable.no  rev_faulted=1 / 3  G_faulted_armature=1e-5 S  fault_trigger_armature=ee.enum.faults.faultTrigger.temporal  t_fault_armature=1 s  max_permissible_current_armature=inf A  t_fail_on_current_armature=1 s  enable_fault_field=ee.enum.faults.faultEnable.no  G_faulted_field=1e-5 S  fault_trigger_field=ee.enum.faults.faultTrigger.temporal  t_fault_field=1 s  max_permissible_current_field=inf A  t_fail_on_current_field=1 s  fault_action=ee.enum.faults.faultAction.none  alpha=3.93e-3 1/K  Tmeas=25 degC  thermal_mass=100 J/K  initial_temperature=25 degC
  Derivative : Derivative
  Electrical Reference : fl_lib/Electrical/Electrical Elements/Electrical Reference
  H-Bridge : ee_lib/Semiconductors & Converters/Converters/H-Bridge  supply_ports=ee.enum.supply_ports.hidesupply  Venable=2.5 V  Vmax=5.0 V  Vreverse=2.5 V  Vbrake=2.5 V  Vm=12 V  pwm_or_av=ee.enum.pwm_or_av.pwm  regenerative_braking_mode=ee.enum.converters.regenerative_braking_mode.depends_on_rev  discontinuous=ee.enum.current_profile.continuous  freewheeling_mode=ee.enum.converters.freewheeling_mode.one_switch_one_diode  Ron=0.1 Ohm  Don=0.05 Ohm  Goff=1e-6 S  Rload=10 Ohm  Lload=1e-5 H  F=10 kHz  thermal_mass=100 J/K  initial_temperature=298.15 K  Ron2=0.1 Ohm  Don2=0.05 Ohm  Tmeas=298.15 K  Tmeas2=398.15 K
  Ideal Rotational Motion Sensor : fl_lib/Mechanical/Mechanical Sensors/Ideal Rotational Motion Sensor  wrap_angle=simscape.enum.onoff.off  offset=0 rad
  J : Gain  Gain=(7.95e-5)
  Mechanical Rotational Reference : fl_lib/Mechanical/Rotational Elements/Mechanical Rotational Reference
  PS-Simulink Converter : nesl_utility/PS-Simulink Converter  PhysicalDomain=network_engine_domain  SubClassName=ps_output  LeftPortType=input  RightPortType=output  PseudoPeriodic=off  Frequencies=[]  Unit=inherit  AffineConversion=off
  Simulink-PS Converter : nesl_utility/Simulink-PS Converter  PhysicalDomain=network_engine_domain  SubClassName=ps_input  LeftPortType=input  RightPortType=output  PseudoPeriodic=off  Frequencies=[]  NoiseDistribution=none  NoiseParameters=[]  Unit=1  AffineConversion=off  FilteringAndDerivatives=provide  SimscapeFilterOrder=1  InputFilterTimeConstant=0.001  UdotUserProvided=0
  Solver Configuration : nesl_utility/Solver Configuration  PhysicalDomain=network_engine_domain  SubClassName=solver  LeftPortType=input  RightPortType=generic  Tones=[]  Harmonics=[]  SimulateNoise=off  Profile=off  UseLocalSampling=off  EnableSwitchedLinearOptims=on  FrequencyDomain=off  UseCCode=off  RelTol=0.001  AbsTol=1e-06  MinStep=1e-09  ToWorkspace=off  RevertToSquareIcSolve=off  NumHomotopyIterations=100  PhasorMode=off  PhasorModeNumHarmonics=1  DoDC=off  ResidualTolerance=1e-09  UseLocalSolver=off  LocalSolverChoice=NE_BACKWARD_EULER_ADVANCER  LocalSolverSampleTime=0.001  DoFixedCost=off  MaxNonlinIter=3  MaxModeIter=2  ComputeImpulses=off  ImpulseIterations=2  LinearAlgebra=auto  EquationFormulation=NE_TIME_EF  DelaysMemoryBudget=1024  AutomaticFiltering=on  FilteringTimeConstant=0.001  PartitionStorageMethod=AS_NEEDED  PartitionMemoryBudget=1024  PartitionMethod=ROBUST
  Sum2 : Sum  Inputs=|++
  b : Gain  Gain=(6.1104e-5)
  Motor torque : Outport
  angular acceleration : Outport  Port=2
  output : Outport  Port=3
  wires:
  Signal1/1 -> Sum2/2
  Signal/1 -> Sum2/1
  Torque_pitch/1 -> Add/3
  Add/1 -> Motor torque/1
  Sum2/1 -> Simulink-PS Converter/1
  b/1 -> Add/2
  Derivative/1 -> angular acceleration/1, J/1
  PS-Simulink Converter/1 -> b/1, output/1, Derivative/1
  J/1 -> Add/1
  connections:
  PS-Simulink Converter/LConn1 -- Ideal Rotational Motion Sensor/RConn2
  H-Bridge/RConn1 -- DC Motor/LConn1
  DC Motor/RConn2 -- Ideal Rotational Motion Sensor/RConn1 -- Mechanical Rotational Reference/LConn1
  Ideal Rotational Motion Sensor/LConn1 -- DC Motor/LConn2
  Controlled PWM Voltage/RConn1 -- H-Bridge/LConn1
  Solver Configuration/RConn1 -- Electrical Reference/LConn1 -- H-Bridge/RConn2 -- DC Motor/RConn1 -- Controlled Voltage Source/RConn2 -- Controlled PWM Voltage/LConn2 -- Controlled PWM Voltage/RConn2 -- H-Bridge/LConn2 -- H-Bridge/LConn3 -- H-Bridge/LConn4
  Simulink-PS Converter/RConn1 -- Controlled Voltage Source/RConn1
  Controlled Voltage Source/LConn1 -- Controlled PWM Voltage/LConn1

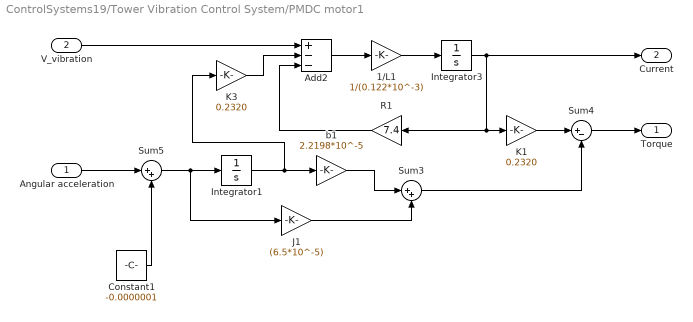
== system ControlSystems19/Tower Vibration Control System/PMDC motor1 ==
  Angular acceleration : Inport
  V_vibration : Inport  Port=2
  1/L1 : Gain  Gain=1/(0.122*10^-3)
  Add2 : Sum  Inputs=+--
  Constant1 : Constant  Value=-0.0000001
  Integrator1 : Integrator
  Integrator3 : Integrator
  J1 : Gain  Gain=(6.5*10^-5)
  K1 : Gain  Gain=0.2320
  K3 : Gain  Gain=0.2320
  R1 : Gain  Gain=7.4
  Sum3 : Sum  Inputs=|++
  Sum4 : Sum  Inputs=|+-
  Sum5 : Sum  Inputs=|++
  b1 : Gain  Gain=2.2198*10^-5
  Torque : Outport
  Current : Outport  Port=2
  wires:
  K3/1 -> Add2/2
  Sum4/1 -> Torque/1
  Add2/1 -> 1/L1/1
  K1/1 -> Sum4/1
  V_vibration/1 -> Add2/1
  Integrator3/1 -> Current/1, R1/1, K1/1
  Constant1/1 -> Sum5/2
  Sum5/1 -> J1/1, Integrator1/1
  Integrator1/1 -> K3/1, b1/1
  1/L1/1 -> Integrator3/1
  b1/1 -> Sum3/1
  Sum3/1 -> Sum4/2
  R1/1 -> Add2/3
  J1/1 -> Sum3/2
  Angular acceleration/1 -> Sum5/1

== system ControlSystems19/Tower Vibration Control System/Subsystem2 ==
  TOW Vibrating acceleration : Inport
  GearRatio : Gain  Gain=1/400
  Angular acceleration : Outport
  wires:
  TOW Vibrating acceleration/1 -> GearRatio/1
  GearRatio/1 -> Angular acceleration/1

== system ControlSystems19/Tower Vibration Control System/Subsystem3 ==
  Torque : Inport
  Raduis : Gain  Gain=4000*0.5
  LInear Force : Outport
  wires:
  Torque/1 -> Raduis/1
  Raduis/1 -> LInear Force/1

== system ControlSystems19/Tower Vibration Control System/Thrust Force2 ==
  v_wind : Inport
  lambda : Inport  Port=2
  beta : Inport  Port=3
  Pi : Gain  Gain=pi
  Product : Product  Inputs=3
  Radius : Constant  Value=35
  Square : Math  Operator=square  SaturateOnIntegerOverflow=on
  Square1 : Math  Operator=square  SaturateOnIntegerOverflow=on
  Subsystem : Subsystem
  half : Gain  Gain=1/2
  F_th : Outport
  wires:
  v_wind/1 -> Square/1
  half/1 -> F_th/1
  Product/1 -> half/1
  Square/1 -> Product/1
  Radius/1 -> Square1/1
  Square1/1 -> Pi/1
  Pi/1 -> Product/2
  lambda/1 -> Subsystem/1(In1)
  beta/1 -> Subsystem/2(In2)
  Subsystem/1(Out1) -> Product/3

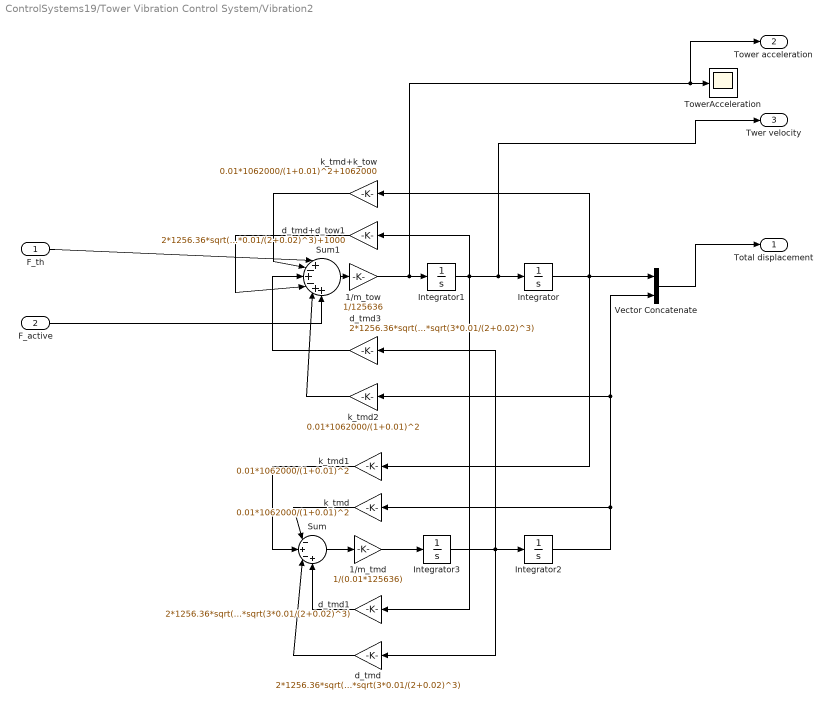
== system ControlSystems19/Tower Vibration Control System/Vibration2 ==
  F_th : Inport
  F_active : Inport  Port=2
  1/m_tmd : Gain  Gain=1/(0.01*125636)
  1/m_tow : Gain  Gain=1/125636
  Integrator : Integrator
  Integrator1 : Integrator  InitialCondition=1.9  UpperSaturationLimit=10  LowerSaturationLimit=-10  AbsoluteTolerance=0.001
  Integrator2 : Integrator
  Integrator3 : Integrator
  Sum : Sum  Inputs=|-+-+
  Sum1 : Sum  Inputs=|+-+-++
  TowerAcceleration : Scope
  Vector Concatenate : Concatenate
  d_tmd : Gain  Gain=2*1256.36*sqrt(1062000/125636)*sqrt(3*0.01/(2+0.02)^3)
  d_tmd+d_tow1 : Gain  Gain=2*1256.36*sqrt(1062000/125636)*sqrt(3*0.01/(2+0.02)^3)+1000
  d_tmd1 : Gain  Gain=2*1256.36*sqrt(1062000/125636)*sqrt(3*0.01/(2+0.02)^3)
  d_tmd3 : Gain  Gain=2*1256.36*sqrt(1062000/125636)*sqrt(3*0.01/(2+0.02)^3)
  k_tmd : Gain  Gain=0.01*1062000/(1+0.01)^2
  k_tmd+k_tow : Gain  Gain=0.01*1062000/(1+0.01)^2+1062000
  k_tmd1 : Gain  Gain=0.01*1062000/(1+0.01)^2
  k_tmd2 : Gain  Gain=0.01*1062000/(1+0.01)^2
  Total displacement : Outport
  Tower acceleration : Outport  Port=2
  Twer velocity : Outport  Port=3
  wires:
  Integrator/1 -> k_tmd+k_tow/1, Vector Concatenate/1, k_tmd1/1
  Integrator3/1 -> d_tmd/1, d_tmd3/1, Integrator2/1
  1/m_tmd/1 -> Integrator3/1
  Sum/1 -> 1/m_tmd/1
  1/m_tow/1 -> Tower acceleration/1, TowerAcceleration/1, Integrator1/1
  Sum1/1 -> 1/m_tow/1
  k_tmd/1 -> Sum/1
  d_tmd/1 -> Sum/3
  d_tmd1/1 -> Sum/4
  k_tmd1/1 -> Sum/2
  k_tmd+k_tow/1 -> Sum1/2
  d_tmd+d_tow1/1 -> Sum1/4
  d_tmd3/1 -> Sum1/3
  Integrator2/1 -> k_tmd/1, k_tmd2/1, Vector Concatenate/2
  k_tmd2/1 -> Sum1/5
  Vector Concatenate/1 -> Total displacement/1
  F_th/1 -> Sum1/1
  F_active/1 -> Sum1/6
  Integrator1/1 -> d_tmd+d_tow1/1, d_tmd1/1, Twer velocity/1, Integrator/1

== system ControlSystems19/Yaw Control System/Aerodynamic Yaw Torque ==
  note: Beta needs to be in radians
  Lambda : Inport
  Yaw Angle radians : Inport  Port=2
  Wind_Vel m/s : Inport  Port=3
  Beta_radians : Inport  Port=4
  Wind Angle radians : Inport  Port=5
  Subtract : Sum  Inputs=+-
  block 1 : Subsystem
  block 2 : Subsystem
  Torque Nm : Outport
  wires:
  block 1/1(C_t) -> block 2/1(Thrust_Coefficient)
  Beta_radians/1 -> block 1/2(beta)
  Wind Angle radians/1 -> Subtract/1
  Yaw Angle radians/1 -> Subtract/2
  Subtract/1 -> block 2/3(Wind Angle difference)
  block 2/1(Yaw_Torque) -> Torque Nm/1
  Lambda/1 -> block 1/1(lambda)
  Wind_Vel m/s/1 -> block 2/2(wind_velocity)

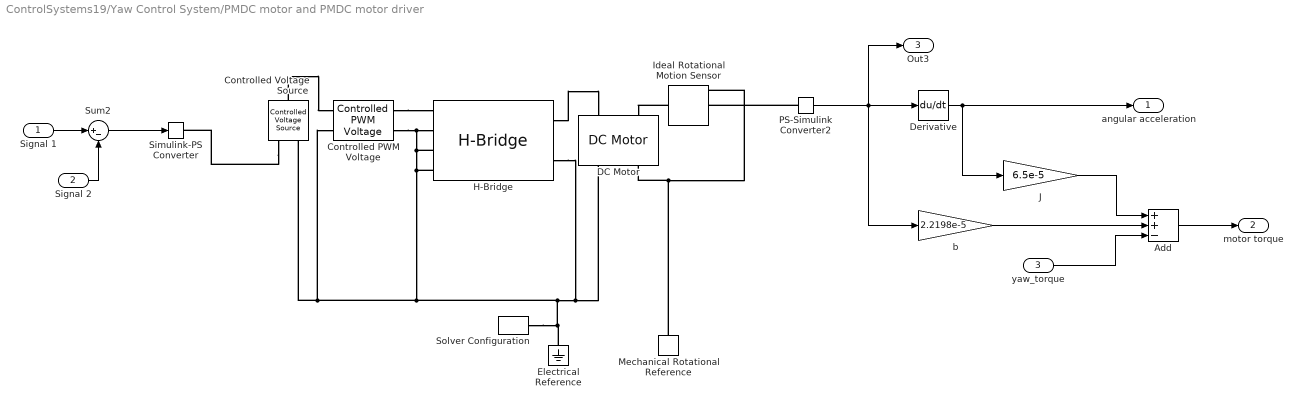
== system ControlSystems19/Yaw Control System/PMDC motor and PMDC motor driver ==
  Signal 1 : Inport
  Signal 2 : Inport  Port=2
  yaw_torque : Inport  Port=3
  Add : Sum  Inputs=++-
  Controlled PWM Voltage : ee_lib/Integrated Circuits/Controlled PWM Voltage  F=1000 Hz  TD=0 s  pulse_width_offset=0 s  pulse_min=0 s  Vmin=0 V  Vmax=5 V  Vm=48 V  pwm_or_av=1  event_type=1  sample_time=1e-6 s  u_min=0  u_max=1
  Controlled Voltage Source : fl_lib/Electrical/Electrical Sources/Controlled Voltage Source
  DC Motor : ee_lib/Electromechanical/Brushed Motors/DC Motor  field_option=ee.enum.field_option.pm  Rf=100 Ohm  Lf=1 H  Laf=0.15 H  If0=0 A  parameterization=ee.enum.dcparam_option.circuit_param  Ra=2.2 Ohm  La=3.343e-3 H  emf_or_torque=ee.enum.emf_or_torque.kv  Kv=0.1183 V/(rad/s)  Ki=6.876e-4 N*m/A  T_stall=0.24e-3 N*m  w_max=19100 rpm  w_rated=15000 rpm  P_rated=0.08 W  V_rated=1.5 V  J=6.5e-5 kg*m^2  lam_param=ee.enum.lam_param.damping  lam=2.2198e-5 N*m/(rad/s)  i_noload=0 A  V_i_noload=1.5 V  speed0=0 rad/s  enable_fault_armature=ee.enum.faults.faultEnable.no  rev_faulted=1 / 3  G_faulted_armature=1e-5 S  fault_trigger_armature=ee.enum.faults.faultTrigger.temporal  t_fault_armature=1 s  max_permissible_current_armature=inf A  t_fail_on_current_armature=1 s  enable_fault_field=ee.enum.faults.faultEnable.no  G_faulted_field=1e-5 S  fault_trigger_field=ee.enum.faults.faultTrigger.temporal  t_fault_field=1 s  max_permissible_current_field=inf A  t_fail_on_current_field=1 s  fault_action=ee.enum.faults.faultAction.none  alpha=3.93e-3 1/K  Tmeas=25 degC  thermal_mass=100 J/K  initial_temperature=25 degC
  Derivative : Derivative
  Electrical Reference : fl_lib/Electrical/Electrical Elements/Electrical Reference
  H-Bridge : ee_lib/Semiconductors & Converters/Converters/H-Bridge  supply_ports=ee.enum.supply_ports.hidesupply  Venable=2.5 V  Vmax=5.0 V  Vreverse=2.5 V  Vbrake=2.5 V  Vm=12 V  pwm_or_av=ee.enum.pwm_or_av.pwm  regenerative_braking_mode=ee.enum.converters.regenerative_braking_mode.depends_on_rev  discontinuous=ee.enum.current_profile.continuous  freewheeling_mode=ee.enum.converters.freewheeling_mode.one_switch_one_diode  Ron=0.1 Ohm  Don=0.05 Ohm  Goff=1e-6 S  Rload=10 Ohm  Lload=1e-5 H  F=10 kHz  thermal_mass=100 J/K  initial_temperature=298.15 K  Ron2=0.1 Ohm  Don2=0.05 Ohm  Tmeas=298.15 K  Tmeas2=398.15 K
  Ideal Rotational Motion Sensor : fl_lib/Mechanical/Mechanical Sensors/Ideal Rotational Motion Sensor  wrap_angle=simscape.enum.onoff.off  offset=0 rad
  J : Gain  Gain=6.5e-5
  Mechanical Rotational Reference : fl_lib/Mechanical/Rotational Elements/Mechanical Rotational Reference
  PS-Simulink Converter2 : nesl_utility/PS-Simulink Converter  PhysicalDomain=network_engine_domain  SubClassName=ps_output  LeftPortType=input  RightPortType=output  PseudoPeriodic=off  Frequencies=[]  Unit=inherit  AffineConversion=off
  Simulink-PS Converter : nesl_utility/Simulink-PS Converter  PhysicalDomain=network_engine_domain  SubClassName=ps_input  LeftPortType=input  RightPortType=output  PseudoPeriodic=off  Frequencies=[]  NoiseDistribution=none  NoiseParameters=[]  Unit=1  AffineConversion=off  FilteringAndDerivatives=provide  SimscapeFilterOrder=1  InputFilterTimeConstant=0.001  UdotUserProvided=0
  Solver Configuration : nesl_utility/Solver Configuration  PhysicalDomain=network_engine_domain  SubClassName=solver  LeftPortType=input  RightPortType=generic  Tones=[]  Harmonics=[]  SimulateNoise=off  Profile=off  UseLocalSampling=off  EnableSwitchedLinearOptims=on  FrequencyDomain=off  UseCCode=off  RelTol=0.001  AbsTol=1e-06  MinStep=1e-09  ToWorkspace=off  RevertToSquareIcSolve=off  NumHomotopyIterations=100  PhasorMode=off  PhasorModeNumHarmonics=1  DoDC=off  ResidualTolerance=1e-09  UseLocalSolver=off  LocalSolverChoice=NE_BACKWARD_EULER_ADVANCER  LocalSolverSampleTime=0.001  DoFixedCost=off  MaxNonlinIter=3  MaxModeIter=2  ComputeImpulses=off  ImpulseIterations=2  LinearAlgebra=auto  EquationFormulation=NE_TIME_EF  DelaysMemoryBudget=1024  AutomaticFiltering=on  FilteringTimeConstant=0.001  PartitionStorageMethod=AS_NEEDED  PartitionMemoryBudget=1024  PartitionMethod=ROBUST
  Sum2 : Sum  Inputs=|+-
  b : Gain  Gain=2.2198e-5
  angular acceleration : Outport
  motor torque : Outport  Port=2
  Out3 : Outport  Port=3
  wires:
  Signal 1/1 -> Sum2/1
  Signal 2/1 -> Sum2/2
  Sum2/1 -> Simulink-PS Converter/1
  yaw_torque/1 -> Add/3
  PS-Simulink Converter2/1 -> Derivative/1, Out3/1, b/1
  Derivative/1 -> J/1, angular acceleration/1
  b/1 -> Add/2
  J/1 -> Add/1
  Add/1 -> motor torque/1
  connections:
  Controlled Voltage Source/RConn1 -- Simulink-PS Converter/RConn1
  Controlled PWM Voltage/RConn1 -- H-Bridge/LConn1
  Ideal Rotational Motion Sensor/LConn1 -- DC Motor/LConn2
  H-Bridge/RConn1 -- DC Motor/LConn1
  Controlled Voltage Source/LConn1 -- Controlled PWM Voltage/LConn1
  Mechanical Rotational Reference/LConn1 -- Ideal Rotational Motion Sensor/RConn1 -- DC Motor/RConn2
  H-Bridge/RConn2 -- Electrical Reference/LConn1 -- Solver Configuration/RConn1 -- H-Bridge/LConn4 -- H-Bridge/LConn3 -- H-Bridge/LConn2 -- Controlled PWM Voltage/RConn2 -- Controlled Voltage Source/RConn2 -- Controlled PWM Voltage/LConn2 -- DC Motor/RConn1
  PS-Simulink Converter2/LConn1 -- Ideal Rotational Motion Sensor/RConn2

== system ControlSystems19/Yaw Control System/Yaw Mechanical System ==
  angular acceleration : Inport
  yaw_aerodynamic_torque : Inport  Port=2
  Add : Sum  Inputs=3
  D_yaw : Gain  Gain=200
  Integrator : Integrator
  Integrator1 : Integrator
  Integrator2 : Integrator
  J_yaw : Gain  Gain=45377
  yaw_angle : Outport
  yaw_torque : Outport  Port=2
  wires:
  Integrator/1 -> yaw_angle/1
  Add/1 -> yaw_torque/1
  D_yaw/1 -> Add/2
  yaw_aerodynamic_torque/1 -> Add/3
  J_yaw/1 -> Add/1
  angular acceleration/1 -> Integrator1/1, J_yaw/1, Integrator2/1
  Integrator1/1 -> D_yaw/1
  Integrator2/1 -> Integrator/1

== system ControlSystems19/Drivetrain/Aerodynamic Block/Power Coefficient ==
  note: http://oaji.net/articles/2017/296-1504711578.pdf
      | Mathematical analysis of tip speed ratio of a wind turbine and its effects on power coefficient
      | Cp = 1/2 ( λ − 0.022β ^2 − 5.6) e −0.17^ λ
  Lamda : Inport
  Beta : Inport  Port=2
  Constant : Constant  Value=5.6
  Exp : Math  SignedPower=on  SaturateOnIntegerOverflow=on
  Gain : Gain  Gain=0.5
  Gain1 : Gain  Gain=0.022
  Gain2 : Gain  Gain=-0.17
  Product : Product
  Square : Math  Operator=square  SaturateOnIntegerOverflow=on
  Sum : Sum  Inputs=|+--
  C_p : Outport
  wires:
  Sum/1 -> Gain/1
  Gain2/1 -> Exp/1
  Constant/1 -> Sum/2
  Gain/1 -> Product/2
  Lamda/1 -> Sum/1, Gain2/1
  Gain1/1 -> Sum/3
  Beta/1 -> Square/1
  Product/1 -> C_p/1
  Exp/1 -> Product/1
  Square/1 -> Gain1/1

== system ControlSystems19/Drivetrain/Aerodynamic Block/Rotor Torque ==
  note: Power of wind
  Power_Coefficient : Inport
  Wind_Speed : Inport  Port=2
  Rotor_Angular_Velocity : Inport  Port=3
  Divide : Product  Inputs=**/
  Gain : Gain  Gain=0.5*1.225*pi*35^2
  Product : Product
  Square : Math  Operator=square  SaturateOnIntegerOverflow=on
  Rotor_Torque : Outport
  wires:
  Rotor_Angular_Velocity/1 -> Divide/3  "omega_rotor"
  Power_Coefficient/1 -> Divide/1
  Divide/1 -> Rotor_Torque/1
  Wind_Speed/1 -> Square/1, Product/1  "V_wind"
  Gain/1 -> Divide/2
  Product/1 -> Gain/1
  Square/1 -> Product/2

== system ControlSystems19/Drivetrain/Aerodynamic Block/Tip speed Ratio ==
  Rotor_Angular_Velocity : Inport
  Wind_Velocity : Inport  Port=2
  Divide : Product  Inputs=*/
  Radius : Gain  Gain=35
  Tip_Speed_Ratio : Outport
  wires:
  Rotor_Angular_Velocity/1 -> Radius/1  "omega_r"
  Radius/1 -> Divide/1
  Wind_Velocity/1 -> Divide/2  "V_wind"
  Divide/1 -> Tip_Speed_Ratio/1

== system ControlSystems19/Drivetrain/Electricl Block/Rotor Reactance ==
  Gain3 : Gain  Gain=2*pi
  Rotor Inductance : Constant  Value=0.000195
  Out1 : Outport
  wires:
  Gain3/1 -> Out1/1
  Rotor Inductance/1 -> Gain3/1

== system ControlSystems19/Drivetrain/Electricl Block/Thevenin Reactance ==
  Divide7 : Product  Inputs=/**
  Magnitude Squared7 : Math  Operator=magnitude^2  SaturateOnIntegerOverflow=on
  Magnitude Squared8 : Math  Operator=magnitude^2  SaturateOnIntegerOverflow=on
  Mutual Reactance : Subsystem
  Product : Product
  Rotor Resistance1 : Constant  Value=0.00763
  Stator Reactance : Subsystem
  Sum1 : Sum  Inputs=|+-
  Sum7 : Sum  Inputs=|++
  Sum8 : Sum  Inputs=|++
  Out1 : Outport
  wires:
  Sum7/1 -> Divide7/1
  Magnitude Squared7/1 -> Sum1/1, Sum7/1
  Divide7/1 -> Out1/1
  Stator Reactance/1(Out1) -> Product/1, Sum8/1
  Sum8/1 -> Product/2, Magnitude Squared8/1
  Rotor Resistance1/1 -> Magnitude Squared7/1
  Magnitude Squared8/1 -> Sum7/2
  Mutual Reactance/1(Out1) -> Divide7/3, Sum8/2
  Sum1/1 -> Divide7/2
  Product/1 -> Sum1/2

== system ControlSystems19/Drivetrain/Electricl Block/Thevenin Resistance ==
  Divide7 : Product  Inputs=**/
  Magnitude Squared6 : Math  Operator=magnitude^2  SaturateOnIntegerOverflow=on
  Magnitude Squared7 : Math  Operator=magnitude^2  SaturateOnIntegerOverflow=on
  Magnitude Squared8 : Math  Operator=magnitude^2  SaturateOnIntegerOverflow=on
  Mutual Reactance : Subsystem
  Rotor Resistance1 : Constant  Value=0.00763
  Stator Reactance : Subsystem
  Sum7 : Sum  Inputs=|++
  Sum8 : Sum  Inputs=|++
  Out1 : Outport
  wires:
  Sum7/1 -> Divide7/3
  Magnitude Squared7/1 -> Sum7/1
  Divide7/1 -> Out1/1
  Stator Reactance/1(Out1) -> Sum8/2
  Sum8/1 -> Magnitude Squared8/1
  Rotor Resistance1/1 -> Divide7/2, Magnitude Squared7/1
  Magnitude Squared6/1 -> Divide7/1
  Magnitude Squared8/1 -> Sum7/2
  Mutual Reactance/1(Out1) -> Sum8/1, Magnitude Squared6/1

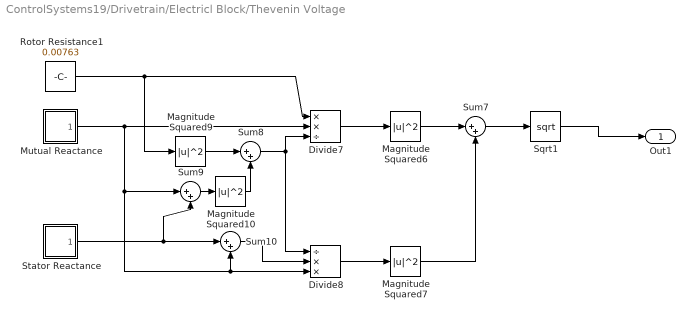
== system ControlSystems19/Drivetrain/Electricl Block/Thevenin Voltage ==
  Divide7 : Product  Inputs=**/
  Divide8 : Product  Inputs=/**
  Magnitude Squared{6..7,9..10} (4 alike) : Math  Operator=magnitude^2  SaturateOnIntegerOverflow=on
  Mutual Reactance : Subsystem
  Rotor Resistance1 : Constant  Value=0.00763
  Sqrt1 : Sqrt  SaturateOnIntegerOverflow=on
  Stator Reactance : Subsystem
  Sum{7..10} (4 alike) : Sum  Inputs=|++
  Out1 : Outport
  wires:
  Sum10/1 -> Divide8/2
  Sum7/1 -> Sqrt1/1
  Sqrt1/1 -> Out1/1
  Mutual Reactance/1(Out1) -> Divide7/2, Sum9/1, Sum10/2, Divide8/3
  Stator Reactance/1(Out1) -> Sum9/2, Sum10/1
  Sum9/1 -> Magnitude Squared10/1
  Magnitude Squared9/1 -> Sum8/1
  Divide8/1 -> Magnitude Squared7/1
  Sum8/1 -> Divide8/1, Divide7/3
  Magnitude Squared10/1 -> Sum8/2
  Magnitude Squared7/1 -> Sum7/2
  Magnitude Squared6/1 -> Sum7/1
  Rotor Resistance1/1 -> Divide7/1, Magnitude Squared9/1
  Divide7/1 -> Magnitude Squared6/1

== system ControlSystems19/Drivetrain/Electricl Block/den ==
  In1 : Inport
  In2 : Inport  Port=2
  Magnitude Squared4 : Math  Operator=magnitude^2  SaturateOnIntegerOverflow=on
  Sum4 : Sum  Inputs=|++
  Out1 : Outport
  wires:
  In2/1 -> Sum4/2
  In1/1 -> Magnitude Squared4/1
  Sum4/1 -> Out1/1
  Magnitude Squared4/1 -> Sum4/1
